simulink subsystem "Trejectory_subsystem"  (R2022b)
settings: Solver=VariableStepAuto  StartTime=0.0  StopTime=10.0  RelTol=1e-3
settings Model: Creator=kevin  LastModifiedBy=kevin

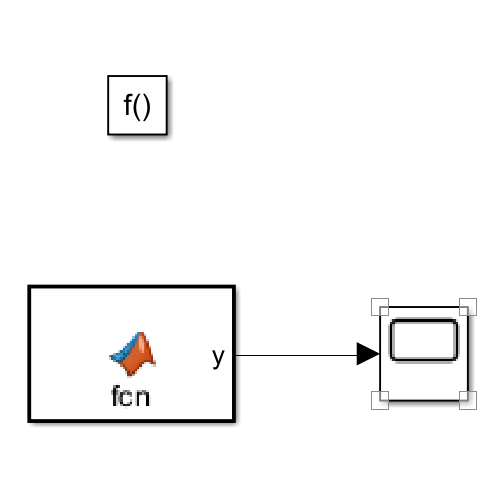
[thumbnail: Simulink's stored preview of the top-level diagram]
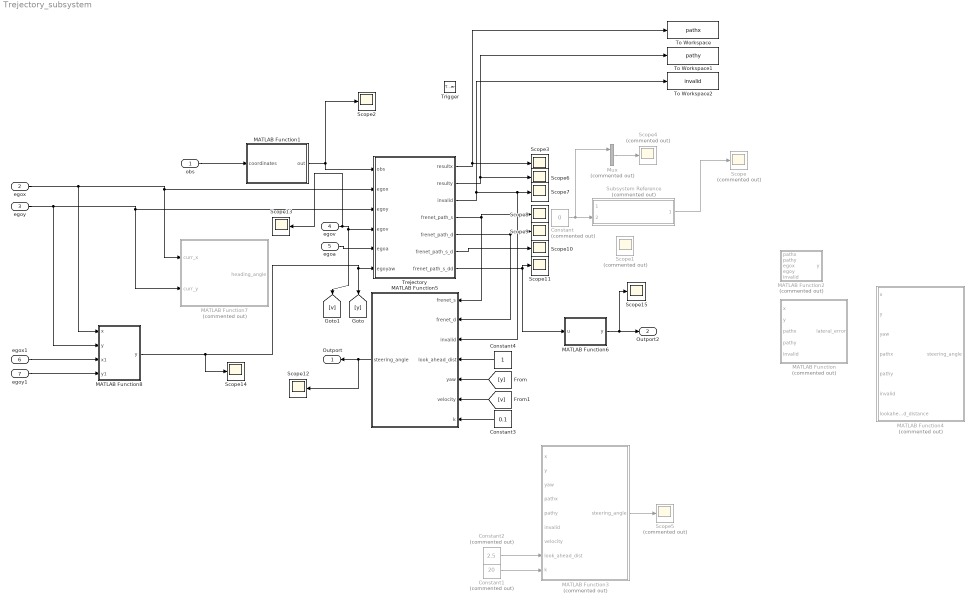
== system Trejectory_subsystem ==
  obs : Inport
  egox : Inport  Port=2
  egoy : Inport  Port=3
  egov : Inport  Port=4
  egoa : Inport  Port=5
  egox1 : Inport  Port=6
  egoy1 : Inport  Port=7
  Trigger : TriggerPort  TriggerType=function-call  VariantControl=(inherit)  PortDimensions=1
  Constant : Constant  Commented=on  Value=0
  Constant1 : Constant  Commented=on  Value=20
  Constant2 : Constant  Commented=on  Value=2.5
  Constant3 : Constant  Value=0.1
  Constant4 : Constant
  MATLAB Function : MATLAB Function  Commented=on  TreatAsAtomicUnit=on
  MATLAB Function1 : MATLAB Function  TreatAsAtomicUnit=on
  MATLAB Function2 : MATLAB Function  Commented=on  TreatAsAtomicUnit=on
  MATLAB Function3 : MATLAB Function  Commented=on  TreatAsAtomicUnit=on
  MATLAB Function4 : MATLAB Function  Commented=on  TreatAsAtomicUnit=on
  MATLAB Function5 : MATLAB Function  TreatAsAtomicUnit=on
  MATLAB Function6 : MATLAB Function  TreatAsAtomicUnit=on
  MATLAB Function7 : MATLAB Function  Commented=on  TreatAsAtomicUnit=on
  MATLAB Function8 : MATLAB Function  TreatAsAtomicUnit=on
  Mux : Mux  Commented=on  Inputs=2
  Scope{,1,4..5} (4 alike) : Scope  Commented=on
  Scope{2..3,6..15} (12 alike) : Scope
  Subsystem Reference : Subsystem  Commented=on  ReferencedSubsystem=PID_controller_subsys
  To Workspace : ToWorkspace  VariableName=pathx  SampleTime=-1
      settings: Save2DSignal=2-D array (concatenate along first dimension)
  To Workspace1 : ToWorkspace  VariableName=pathy  SampleTime=-1
      settings: Save2DSignal=2-D array (concatenate along first dimension)
  To Workspace2 : ToWorkspace  VariableName=invalid  SampleTime=-1
      settings: Save2DSignal=2-D array (concatenate along first dimension)
  Trejectory : MATLAB Function  TreatAsAtomicUnit=on
  Outport : Outport
  Outport2 : Outport  Port=2
  wires:
  MATLAB Function1/1(out) -> Trejectory/1(obs), Scope2/1
  obs/1 -> MATLAB Function1/1(coordinates)
  egox/1 -> Trejectory/2(egox), MATLAB Function7/1(curr_x), MATLAB Function8/1(x)
  egoy/1 -> Trejectory/3(egoy), MATLAB Function7/2(curr_y), MATLAB Function8/2("y ")
  egov/1 -> [v], Trejectory/4(egov), Scope13/1
  egoa/1 -> Trejectory/5(egoa)
  Subsystem Reference/1 -> Scope/1
  Constant/1 -> Subsystem Reference/2, Mux/1
  Mux/1 -> Scope4/1
  MATLAB Function3/1(steering_angle) -> Scope5/1
  Constant1/1 -> MATLAB Function3/9(k)
  Constant2/1 -> MATLAB Function3/8(look_ahead_dist)
  Trejectory/1(resultx) -> Scope3/1, To Workspace/1
  Trejectory/2(resulty) -> Scope6/1, To Workspace1/1
  Trejectory/3(invalid) -> To Workspace2/1, Scope7/1, MATLAB Function5/3(invalid)
  Trejectory/4(frenet_path_s) -> MATLAB Function5/1(frenet_s), Scope8/1
  Trejectory/5(frenet_path_d) -> MATLAB Function5/2(frenet_d), Scope9/1
  Trejectory/6(frenet_path_s_d) -> Scope10/1
  Trejectory/7(frenet_path_s_dd) -> MATLAB Function6/1(u), Scope11/1
  [y] -> MATLAB Function5/5(yaw)
  [v] -> MATLAB Function5/6(velocity)
  Constant3/1 -> MATLAB Function5/7(k)
  MATLAB Function5/1(steering_angle) -> Outport/1, Scope12/1
  MATLAB Function6/1(y) -> Outport2/1, Scope15/1
  Constant4/1 -> MATLAB Function5/4(look_ahead_dist)
  egox1/1 -> MATLAB Function8/3(x1)
  egoy1/1 -> MATLAB Function8/4(y1)
  MATLAB Function8/1(y) -> Trejectory/6(egoyaw), [y], Scope14/1

== matlab function Trejectory_subsystem/MATLAB Function5 ==
  data: frenet_s input; steering_angle output; frenet_d input; invalid input; look_ahead_dist input; yaw input; velocity input; k input
function steering_angle = stanley_control(frenet_s, frenet_d,invalid, look_ahead_dist, yaw, velocity,k)
    valid_indices = find(invalid > 0);
    if isempty(valid_indices) || length(valid_indices) <= 1
        steering_angle = yaw;
        return
    end

    localPoints = zeros(length(valid_indices),2);
    localPoints(:,1) = frenet_s(valid_indices);
    localPoints(:,2) = frenet_d(valid_indices);

    polyFit = PolynomialFitting_class(5, length(valid_indices),1e-2);
    polyFit = polyFit.fit(localPoints);
    limit = 0.5;
%     y_look_ahead = polyFit.evaluate(look_ahead_dist);
%     dy_look_ahead = polyFit.differentiate(look_ahead_dist);
    y_look_ahead = polyFit.evaluate(localPoints(end,1));
    dy_look_ahead = polyFit.differentiate(localPoints(end,1));
    epsilon = 0.01;
    
    steering_angle = dy_look_ahead + atan2(k*y_look_ahead,velocity+epsilon);
    %steering_angle = yaw + atan2(k*localPoints(1,2),velocity+epsilon);
    if abs(steering_angle) > limit
        steering_angle = limit*steering_angle/abs(steering_angle);
    end
end

== matlab function Trejectory_subsystem/MATLAB Function6 ==
  data: u input; y output
function y = fcn(u)

    y = u(6);
end

== matlab function Trejectory_subsystem/MATLAB Function7 ==
  data: curr_x input; heading_angle output; curr_y input
function heading_angle = calc_heading_angle(curr_x, curr_y)
    % Calculate the heading angle based on previous and current positions
    persistent prev_x prev_y;
    
    % Initialize previous coordinates if they don't exist
    if isempty(prev_x)
        prev_x = curr_x;
        prev_y = curr_y;
        heading_angle = 0;
        return;
    end
    
    dx = curr_x - prev_x;
    dy = curr_y - prev_y;
    
    heading_angle = atan2(dy, dx);
    
    % Update previous coordinates for the next iteration
    prev_x = curr_x;
    prev_y = curr_y;
end

== matlab function Trejectory_subsystem/MATLAB Function8 ==
  data: x input; y output; y input; x1 input; y1 input
function y = fcn(x,y,x1,y1)
    y = atan2(y1-y,x1-x);
end

== matlab function Trejectory_subsystem/MATLAB Function1 ==
  data: coordinates input; out output
function out = processCoordinates(coordinates)
    % coordinates 배열에서 x와 y 좌표를 분리하여 처리
    out = zeros(length(coordinates)/2,2);
    out(:,1) = coordinates(1:length(coordinates)/2);
    out(:,2) = coordinates(length(coordinates)/2+1:length(coordinates));
%     out(1,1) = -30.0897;
%     out(1,2) = 20.7625;
end

== matlab function Trejectory_subsystem/Trejectory ==
  data: resultx output; obs input; egox input; egoy input; egov input; egoa input; egoyaw input; resulty output; invalid output; frenet_path_s output; frenet_path_d output; frenet_path_s_d output; frenet_path_s_dd output
function [resultx,resulty,invalid,frenet_path_s, frenet_path_d, frenet_path_s_d, frenet_path_s_dd] = fcn(obs,egox,egoy,egov,egoa,egoyaw)
%function [frenet_path_s, frenet_path_d, frenet_path_s_d, frenet_path_s_dd,opt_d] = Trejectory_function2(obs_global, global_x, global_y, local_v, local_a, local_yaw,opt_d_prev)
    [resultx,resulty,invalid,frenet_path_s, frenet_path_d, frenet_path_s_d, frenet_path_s_dd] = Trejectory_function(obs,egox,egoy,egov,egoa,egoyaw);
    %[pathx,pathy] = Copy_of_Trejectory_function(obs,egox,egoy,egov,egoa);
    %[frenet_path_s, frenet_path_d, frenet_path_s_d, frenet_path_s_dd,opt_d] = Trejectory_function2(obs_global, global_x, global_y, local_v, local_a, local_yaw,opt_d_prev);

end

== matlab function Trejectory_subsystem/MATLAB Function2 ==
  data: pathx input; pathy input; y output; egox input; egoy input; invalid input
function y = fcn(pathx,pathy,egox,egoy,invalid)
    y = calculate_reference(pathx,pathy,egox,egoy,invalid);
end

== matlab function Trejectory_subsystem/MATLAB Function ==
  data: x input; lateral_error output; y input; pathx input; pathy input; invalid input
function lateral_error = calc_lateral_error(x, y, pathx, pathy,invalid)
    % 현재 차량 위치에서 가장 가까운 경로 상의 점 찾기
    valid_indices = find(invalid > 0);
    path_x = pathx(valid_indices);
    path_y = pathy(valid_indices);

    nearest_x = path_x(2);
    nearest_y = path_y(2);
    
    % 횡방향 오차 계산
    path_vector = [path_x(2+1) - nearest_x, path_y(2+1) - nearest_y];
    vehicle_vector = [x - nearest_x, y - nearest_y];
    lateral_error = norm(cross([path_vector 0], [vehicle_vector 0])) / norm(path_vector);
    
    % 횡방향 오차의 부호 결정
    cross_product = cross([path_vector 0], [vehicle_vector 0]);
    if cross_product(3) < 0
        lateral_error = -lateral_error;
    end
end

== matlab function Trejectory_subsystem/MATLAB Function3 ==
  data: x input; steering_angle output; y input; yaw input; pathx input; pathy input; invalid input; velocity input; look_ahead_dist input; k input
function steering_angle = stanley_control(x, y, yaw, pathx, pathy,invalid,velocity,look_ahead_dist,k)
    valid_indices = find(invalid > 0);
    if isempty(valid_indices) || length(valid_indices) <= 1
        steering_angle = yaw;
        return
    end
%     path_x = pathx(valid_indices);
%     path_y = pathy(valid_indices);
    path_x = pathx(2);
    path_y = pathy(2);
    frenet_x = (x - path_x) * cos(yaw) + (y - path_y) * sin(yaw);
    frenet_y = -(x - path_x) * sin(yaw) + (y - path_y) * cos(yaw);

%     localPoints = zeros(length(valid_indices),2);
%     localPoints(:,1) = frenet_x;
%     localPoints(:,2) = frenet_y;
% 
%     polyFit = PolynomialFitting_class(length(valid_indices)-1, length(valid_indices),1e-1);
%     polyFit = polyFit.fit(localPoints);
% 
%     y_look_ahead = polyFit.evaluate(look_ahead_dist);
%     dy_look_ahead = polyFit.differentiate(look_ahead_dist);
    y_look_ahead = frenet_y;
    dy_look_ahead = frenet_y/frenet_x;
    epsilon = 0.001;

    steering_angle = dy_look_ahead + atan(k*y_look_ahead/velocity+epsilon);

end

== matlab function Trejectory_subsystem/MATLAB Function4 ==
  data: x input; steering_angle output; y input; yaw input; pathx input; pathy input; invalid input; lookahead_distance input
function steering_angle = pure_pursuit_control(x, y, yaw, pathx, pathy,invalid, lookahead_distance)
    % 차량의 현재 위치에서 가장 가까운 경로 상의 점 찾기
    valid_indices = find(invalid > 0);
    path_x = pathx(valid_indices);
    path_y = pathy(valid_indices);

    distances = sqrt((path_x - x).^2 + (path_y - y).^2);
    [~, min_index] = min(distances);
    
    % 경로 상의 목표 지점 선택
    lookahead_index = min_index;
    while lookahead_index < length(path_x) && distances(lookahead_index) < lookahead_distance
        lookahead_index = lookahead_index + 1;
    end
    
    if lookahead_index >= length(path_x)
        lookahead_index = length(path_x);
    end
    
    target_x = path_x(lookahead_index);
    target_y = path_y(lookahead_index);
    
    % 차량 좌표계에서의 목표 지점 계산
    dx = target_x - x;
    dy = target_y - y;
    target_distance = sqrt(dx^2 + dy^2);
    
    target_local_x = dx * cos(yaw) + dy * sin(yaw);
    target_local_y = -dx * sin(yaw) + dy * cos(yaw);
    
    % 조향각 계산
    steering_angle = atan2(2 * target_local_y * lookahead_distance, target_distance^2);
end
